simulink model "Project1"  (R2014a)
settings: Solver=ode3  StartTime=0.0  StopTime=30  FixedStep=0.01  RelTol=1e-3
settings Model: Creator=dzr3qn  LastModifiedBy=DZR3QN

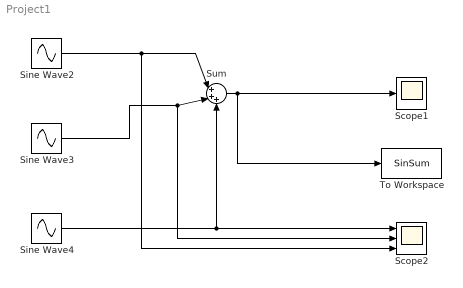
== system Project1 ==
  Scope1 : Scope
  Scope2 : Scope  NumInputPorts=3
      settings: YMin=-5~-5~-5  YMax=5~5~5  SaveName=ScopeData2
  Sine Wave2 : Sin  SampleTime=0
  Sine Wave3 : Sin  Frequency=5  SampleTime=0
  Sine Wave4 : Sin  Frequency=10  SampleTime=0
  Sum : Sum  Inputs=|+++
  To Workspace : ToWorkspace  VariableName=SinSum  SaveFormat=Timeseries  SampleTime=-1
  wires:
  Sum/1 -> To Workspace/1, Scope1/1
  Sine Wave2/1 -> Scope2/3, Sum/1
  Sine Wave3/1 -> Scope2/2, Sum/2
  Sine Wave4/1 -> Sum/3, Scope2/1
